simulink model "Project_4_Model"  (R2024b)
settings: Solver=ode4  StartTime=0.0  StopTime=3600  FixedStep=time_step  RelTol=1e-3
undefined symbols (not defined in the file or in its folder): datBat, datCar, datMotor
settings Model: SimulationMode=accelerator  Creator=andis  LastModifiedBy=tyler

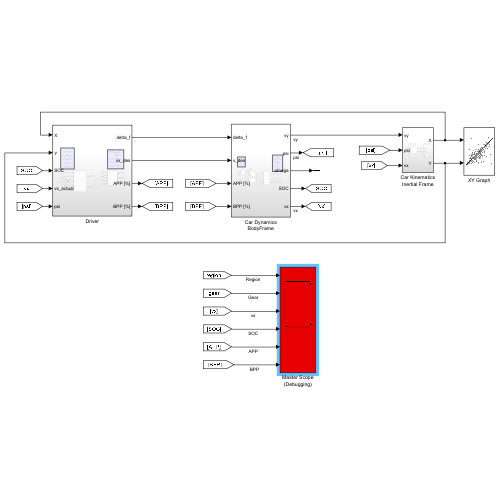
[thumbnail: Simulink's stored preview of the top-level diagram]
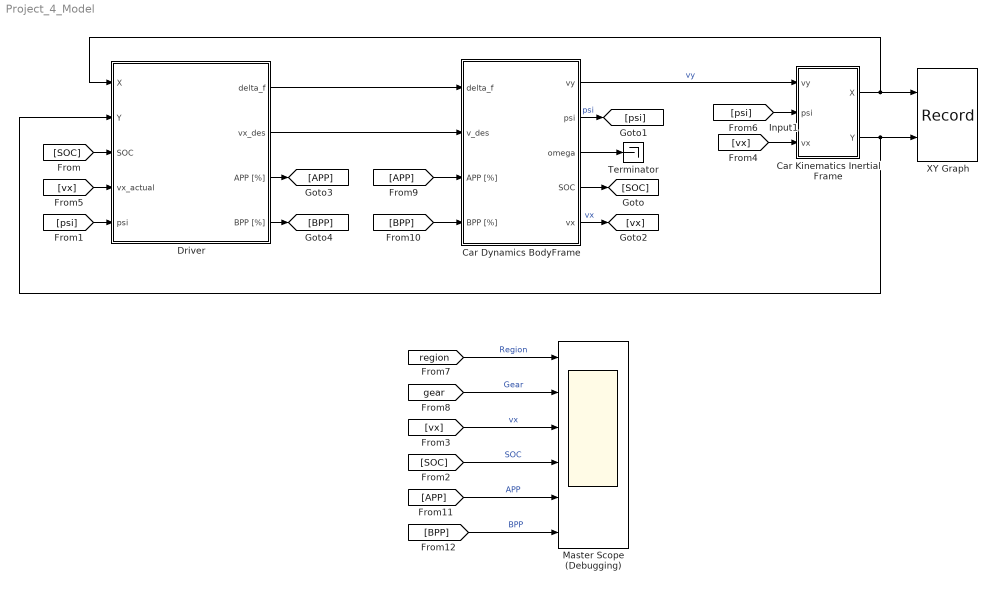
== system Project_4_Model ==
  Input1 : Inport
  Car Dynamics BodyFrame : Subsystem
  Car Kinematics Inertial Frame : Subsystem
  Driver : Subsystem
  Master Scope (Debugging) : Scope  NumInputPorts=6
  Terminator : Terminator
  XY Graph : Record  FileSettingsInternal="{\"entries\":[{\"content\":{\"excelSettings\":{\"content\":{},\"type\":\"Streamout.ExcelSettings\"}},\"type\":\"Streamout.FileSettingStorage\",\"uuid\":\"\"}],\"packageUris\":[\"http:\\/\\/schema.mathworks.com\\/mf0\\/streamout_blocks\\/R2020a\"],\"version\":\"1.0\"}"  Layout=[1 1]  SignalsInternal="{\"entries\":[{\"content\":{\"signals\":[{\"content\":{\"blockPath\":[],\"dimensions\":[1],\"domain\":\"\",\"lineColor\":\"#64d413\",\"lineWidth\":2,\"plots\":[ 1 ],\"port\":1,\"sid\":[\"\"],\"signalID\":1,\"signalName\":\"Car Kinematics\\nInertial Frame:1\"},\"type\":\"RecordBlkView.Signal\",\"uuid\":\"\"},{\"content\":{\"blockPath\":[],\"dimensions\":[1],\"domain\":\"\",\"lineColor\":\"#ff13a6\",\"lineWidth\":2,\"plots\":[ 1 ],\"port\":2,\"sid\":[\"\"],\"signalID\":2,\"signalName\":\"Car Kinematics\\nInertial Frame:2\"},\"type\":\"RecordBlkView.Signal\",\"uuid\":\"\"}]},\"type\":\"RecordBlkView.InputSignals\",\"uuid\":\"\"}],\"packageUris\":[\"http:\\/\\/schema.mathworks.com\\/mf0\\/streamout_blocks\\/R2020a\"],\"version\":\"1.0\"}"  VisualizationBindings="{\"xyplotplugin\":{\"info\":[{\"series\":[{\"bindingParametersList\":[{\"parameter\":\"X-Axis\",\"signalID\":1,\"signalName\":\"Car Kinematics\\nInertial Frame:1\"},{\"parameter\":\"Y-Axis\",\"signalID\":2,\"signalName\":\"Car Kinematics\\nInertial Frame:2\"}],\"seriesID\":0}],\"subplotID\":1}]}}"  CompatibilityTag=XY
  wires:
  Driver/1(delta_f) -> Car Dynamics BodyFrame/1(delta_f)
  Driver/2(vx_des) -> Car Dynamics BodyFrame/2(v_des)
  Car Dynamics BodyFrame/1(vy) -> Car Kinematics Inertial Frame/1(vy)  "vy"
  Car Kinematics Inertial Frame/1(X) -> XY Graph/1, Driver/1(X)
  Car Kinematics Inertial Frame/2(Y) -> Driver/2(Y), XY Graph/2
  Car Dynamics BodyFrame/3(omega) -> Terminator/1
  Car Dynamics BodyFrame/4(SOC) -> [SOC]
  [SOC] -> Driver/3(SOC)
  [psi] -> Driver/5(psi)
  Car Dynamics BodyFrame/2(psi) -> [psi]  "psi"
  [SOC] -> Master Scope (Debugging)/4  "SOC"
  [vx] -> Master Scope (Debugging)/3  "vx"
  [region] -> Master Scope (Debugging)/1  "Region"
  Car Dynamics BodyFrame/5(vx) -> [vx]  "vx"
  [vx] -> Car Kinematics Inertial Frame/3(vx)
  [vx] -> Driver/4(vx_actual)
  [psi] -> Car Kinematics Inertial Frame/2(psi)
  [gear] -> Master Scope (Debugging)/2  "Gear"
  Driver/3(APP [%]) -> [APP]
  Driver/4(BPP [%]) -> [BPP]
  [APP] -> Car Dynamics BodyFrame/3(APP [%])
  [BPP] -> Car Dynamics BodyFrame/4(BPP [%])
  [APP] -> Master Scope (Debugging)/5  "APP"
  [BPP] -> Master Scope (Debugging)/6  "BPP"

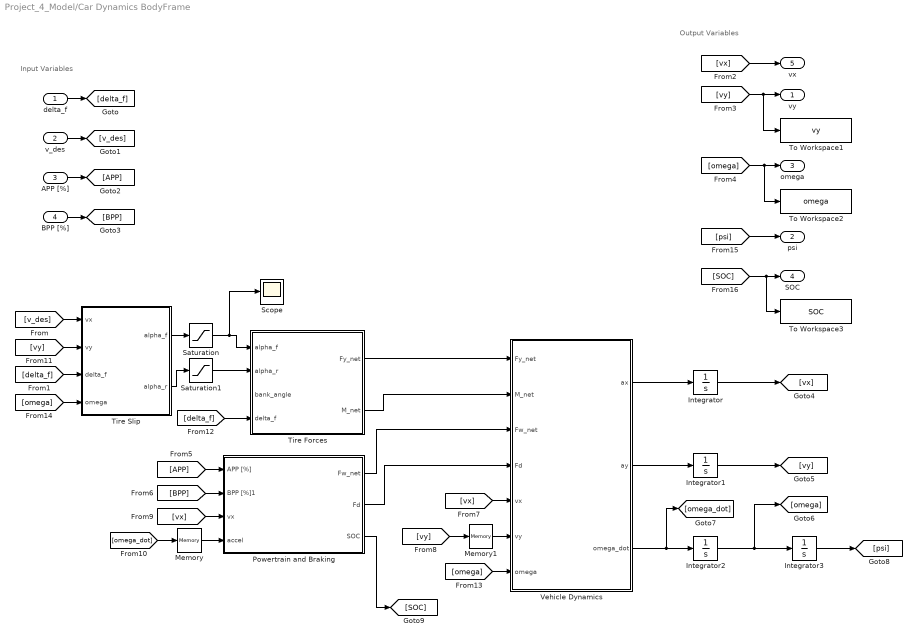
== system Project_4_Model/Car Dynamics BodyFrame ==
  note: Output Variables
  note: Input Variables
  delta_f : Inport
  v_des : Inport  Port=2
  APP [%] : Inport  Port=3
  BPP [%] : Inport  Port=4
  Integrator{,1..3} (4 alike) : Integrator
  Memory : Memory
  Memory1 : Memory
  Powertrain and Braking : Subsystem
  Saturation : Saturate
  Saturation1 : Saturate
  Scope : Scope
  Tire Forces : MATLAB Function  TreatAsAtomicUnit=on
  Tire Slip : MATLAB Function  TreatAsAtomicUnit=on
  To Workspace1 : ToWorkspace  VariableName=vy  SaveFormat=Timeseries  SampleTime=-1
  To Workspace2 : ToWorkspace  VariableName=omega  SaveFormat=Timeseries  SampleTime=-1
  To Workspace3 : ToWorkspace  VariableName=SOC  SaveFormat=Timeseries  SampleTime=-1
  Vehicle Dynamics : MATLAB Function  TreatAsAtomicUnit=on
  vy : Outport
  psi : Outport  Port=2
  omega : Outport  Port=3
  SOC : Outport  Port=4
  vx : Outport  Port=5
  wires:
  Tire Forces/1(Fy_net) -> Vehicle Dynamics/1(Fy_net)
  Tire Forces/2(M_net) -> Vehicle Dynamics/2(M_net)
  delta_f/1 -> [delta_f]
  v_des/1 -> [v_des]
  APP [%]/1 -> [APP]
  BPP [%]/1 -> [BPP]
  [v_des] -> Tire Slip/1(vx)
  [delta_f] -> Tire Slip/3(delta_f)
  Vehicle Dynamics/1(ax) -> Integrator/1
  Vehicle Dynamics/2(ay) -> Integrator1/1
  Vehicle Dynamics/3(omega_dot) -> Integrator2/1, [omega_dot]
  Integrator/1 -> [vx]
  Integrator1/1 -> [vy]
  Integrator2/1 -> [omega], Integrator3/1
  [vx] -> vx/1
  [vy] -> vy/1, To Workspace1/1
  [omega] -> To Workspace2/1, omega/1
  [BPP] -> Powertrain and Braking/2(BPP [%]1)
  [APP] -> Powertrain and Braking/1(APP [%])
  Powertrain and Braking/1(Fw_net) -> Vehicle Dynamics/3(Fw_net)
  Powertrain and Braking/2(Fd) -> Vehicle Dynamics/4(Fd)
  [vx] -> Vehicle Dynamics/5(vx)
  [vx] -> Powertrain and Braking/3(vx)
  [omega_dot] -> Memory/1
  [vy] -> Tire Slip/2(vy)
  [delta_f] -> Tire Forces/4(delta_f)
  Tire Slip/2(alpha_r) -> Saturation1/1
  Tire Slip/1(alpha_f) -> Saturation/1
  Saturation/1 -> Scope/1, Tire Forces/1(alpha_f)
  Saturation1/1 -> Tire Forces/2(alpha_r)
  [omega] -> Vehicle Dynamics/7(omega)
  [omega] -> Tire Slip/4(omega)
  [psi] -> psi/1
  [SOC] -> To Workspace3/1, SOC/1
  Powertrain and Braking/3(SOC) -> [SOC]
  Memory/1 -> Powertrain and Braking/4(accel)
  Integrator3/1 -> [psi]
  Memory1/1 -> Vehicle Dynamics/6(vy)
  [vy] -> Memory1/1

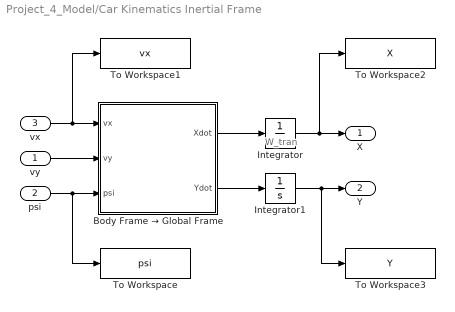
== system Project_4_Model/Car Kinematics Inertial Frame ==
  note: W_tran
  vy : Inport
  psi : Inport  Port=2
  vx : Inport  Port=3
  Body Frame → Global Frame : MATLAB Function  TreatAsAtomicUnit=on
  Integrator : Integrator
  Integrator1 : Integrator
  To Workspace : ToWorkspace  VariableName=psi  SaveFormat=Timeseries  SampleTime=-1
  To Workspace1 : ToWorkspace  VariableName=vx  SaveFormat=Timeseries  SampleTime=-1
  To Workspace2 : ToWorkspace  VariableName=X  SaveFormat=Timeseries  SampleTime=-1
  To Workspace3 : ToWorkspace  VariableName=Y  SaveFormat=Timeseries  SampleTime=-1
  X : Outport
  Y : Outport  Port=2
  wires:
  psi/1 -> To Workspace/1, Body Frame → Global Frame/3(psi)
  Body Frame → Global Frame/1(Xdot) -> Integrator/1
  Body Frame → Global Frame/2(Ydot) -> Integrator1/1
  Integrator1/1 -> To Workspace3/1, Y/1
  Integrator/1 -> To Workspace2/1, X/1
  vx/1 -> To Workspace1/1, Body Frame → Global Frame/1(vx)
  vy/1 -> Body Frame → Global Frame/2(vy)

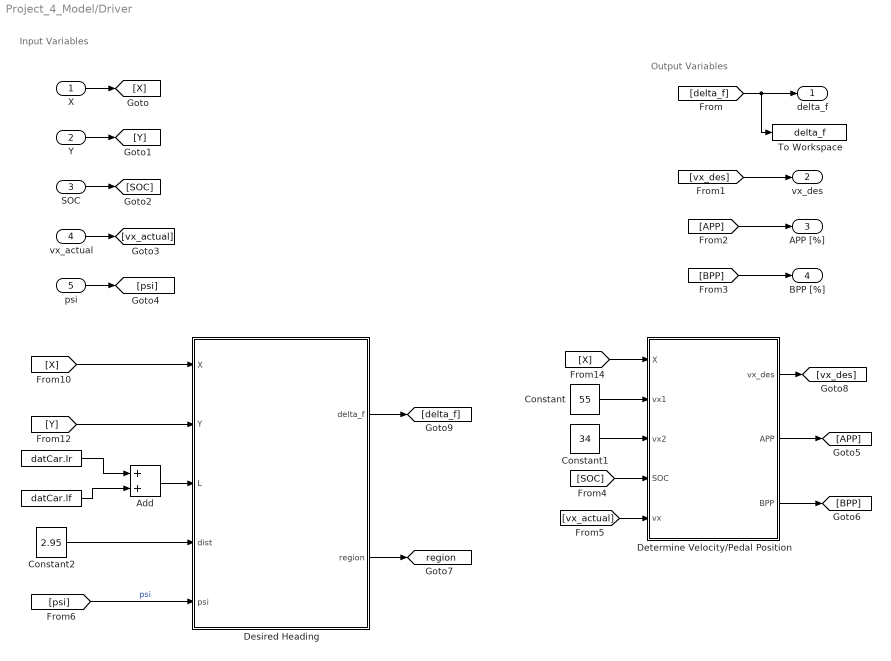
== system Project_4_Model/Driver ==
  note: Output Variables
  note: Input Variables
  X : Inport
  Y : Inport  Port=2
  SOC : Inport  Port=3
  vx_actual : Inport  Port=4
  psi : Inport  Port=5
  " " : Constant  Value=datCar.lr
  "  " : Constant  Value=datCar.lf
  Add : Sum
  Constant : Constant  Value=55
  Constant1 : Constant  Value=34
  Constant2 : Constant  Value=2.95
  Desired Heading : MATLAB Function  TreatAsAtomicUnit=on
  Determine Velocity/Pedal Position : MATLAB Function  TreatAsAtomicUnit=on
  To Workspace : ToWorkspace  VariableName=delta_f  SaveFormat=Timeseries  SampleTime=-1
  delta_f : Outport
  vx_des : Outport  Port=2
  APP [%] : Outport  Port=3
  BPP [%] : Outport  Port=4
  tag scope: region=global
  wires:
  X/1 -> [X]
  Y/1 -> [Y]
  SOC/1 -> [SOC]
  [delta_f] -> To Workspace/1, delta_f/1
  [vx_des] -> vx_des/1
  [APP] -> APP [%]/1
  [BPP] -> BPP [%]/1
  Constant1/1 -> Determine Velocity/Pedal Position/3(vx2)
  Constant/1 -> Determine Velocity/Pedal Position/2(vx1)
  [X] -> Desired Heading/1(X)
  [Y] -> Desired Heading/2(Y)
  [X] -> Determine Velocity/Pedal Position/1(X)
  Determine Velocity/Pedal Position/1(vx_des) -> [vx_des]
  Determine Velocity/Pedal Position/2(APP) -> [APP]
  Determine Velocity/Pedal Position/3(BPP) -> [BPP]
  [SOC] -> Determine Velocity/Pedal Position/4(SOC)
  vx_actual/1 -> [vx_actual]
  [vx_actual] -> Determine Velocity/Pedal Position/5(vx)
  Add/1 -> Desired Heading/3(L)
  "  "/1 -> Add/2
  " "/1 -> Add/1
  Desired Heading/1(delta_f) -> [delta_f]
  Constant2/1 -> Desired Heading/4(dist)
  psi/1 -> [psi]
  [psi] -> Desired Heading/5(psi)  "psi"
  Desired Heading/2(region) -> [region]

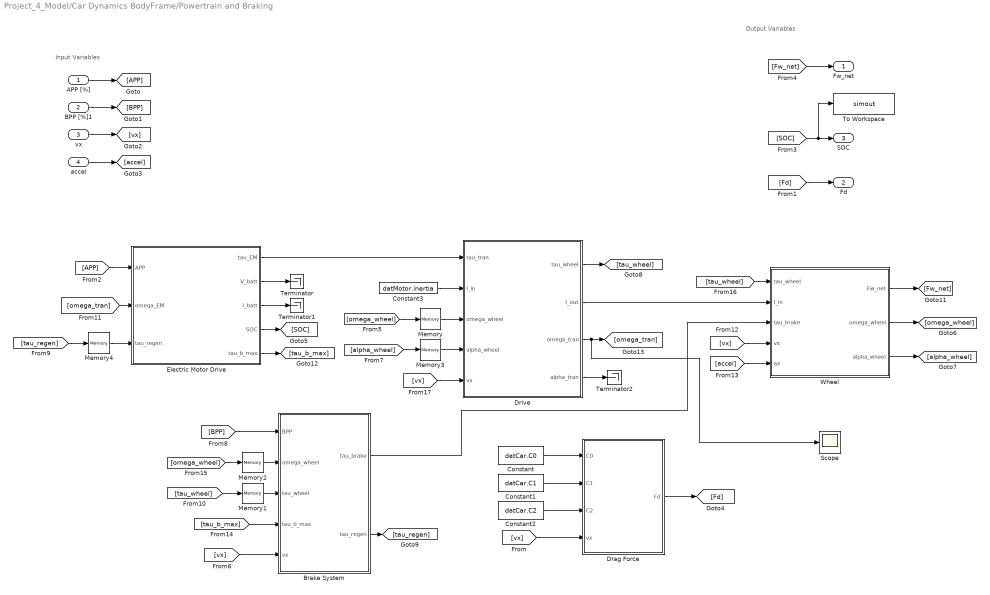
== system Project_4_Model/Car Dynamics BodyFrame/Powertrain and Braking ==
  note: Output Variables
  note: Input Variables
  APP [%] : Inport
  BPP [%]1 : Inport  Port=2
  vx : Inport  Port=3
  accel : Inport  Port=4
  Brake System : Subsystem
  Constant : Constant  Value=datCar.C0
  Constant1 : Constant  Value=datCar.C1
  Constant2 : Constant  Value=datCar.C2
  Constant3 : Constant  Value=datMotor.inertia
  Drag Force : MATLAB Function  TreatAsAtomicUnit=on
  Drive : Subsystem
  Electric Motor Drive : Subsystem
  Memory{,1..4} (5 alike) : Memory
  Scope : Scope
  Terminator : Terminator
  Terminator1 : Terminator
  Terminator2 : Terminator
  To Workspace : ToWorkspace  VariableName=simout  SaveFormat=Timeseries  SampleTime=-1
  Wheel : Subsystem
  Fw_net : Outport
  Fd : Outport  Port=2
  SOC : Outport  Port=3
  wires:
  APP [%]/1 -> [APP]
  BPP [%]1/1 -> [BPP]
  vx/1 -> [vx]
  accel/1 -> [accel]
  Constant/1 -> Drag Force/1(C0)
  Constant1/1 -> Drag Force/2(C1)
  Constant2/1 -> Drag Force/3(C2)
  [vx] -> Drag Force/4(vx)
  Drag Force/1(Fd) -> [Fd]
  [Fd] -> Fd/1
  [APP] -> Electric Motor Drive/1(APP)
  [SOC] -> To Workspace/1, SOC/1
  [Fw_net] -> Fw_net/1
  Electric Motor Drive/4(SOC) -> [SOC]
  Electric Motor Drive/2(V_batt) -> Terminator/1
  Electric Motor Drive/3(I_batt) -> Terminator1/1
  Electric Motor Drive/1(tau_EM) -> Drive/1(tau_tran)
  Wheel/2(omega_wheel) -> [omega_wheel]
  [omega_wheel] -> Memory/1
  [omega_wheel] -> Memory2/1
  Wheel/3(alpha_wheel) -> [alpha_wheel]
  [alpha_wheel] -> Memory3/1
  [BPP] -> Brake System/1(BPP)
  Drive/1(tau_wheel) -> [tau_wheel]
  [tau_wheel] -> Memory1/1
  Drive/2(I_out) -> Wheel/2(I_in)
  Brake System/1(tau_brake) -> Wheel/3(tau_brake)
  Drive/4(alpha_tran) -> Terminator2/1
  Drive/3(omega_tran) -> Scope/1, [omega_tran]
  [omega_tran] -> Electric Motor Drive/2(omega_EM)
  [vx] -> Wheel/4(vx)
  Wheel/1(Fw_net) -> [Fw_net]
  [accel] -> Wheel/5(ax)
  Constant3/1 -> Drive/2(I_in)
  [tau_b_max] -> Brake System/4(tau_b_max)
  Electric Motor Drive/5(tau_b_max) -> [tau_b_max]
  [vx] -> Brake System/5(vx)
  Brake System/2(tau_regen) -> [tau_regen]
  [tau_regen] -> Memory4/1
  Memory/1 -> Drive/3(omega_wheel)
  Memory1/1 -> Brake System/3(tau_wheel)
  Memory2/1 -> Brake System/2(omega_wheel)
  Memory3/1 -> Drive/4(alpha_wheel)
  Memory4/1 -> Electric Motor Drive/3(tau_regen)
  [tau_wheel] -> Wheel/1(tau_wheel)
  [vx] -> Drive/5(vx)

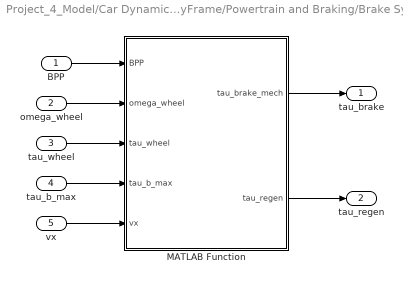
== system Project_4_Model/Car Dynamics BodyFrame/Powertrain and Braking/Brake System ==
  BPP : Inport
  omega_wheel : Inport  Port=2
  tau_wheel : Inport  Port=3
  tau_b_max : Inport  Port=4
  vx : Inport  Port=5
  MATLAB Function : MATLAB Function  TreatAsAtomicUnit=on
  tau_brake : Outport
  tau_regen : Outport  Port=2
  wires:
  BPP/1 -> MATLAB Function/1(BPP)
  omega_wheel/1 -> MATLAB Function/2(omega_wheel)
  tau_wheel/1 -> MATLAB Function/3(tau_wheel)
  tau_b_max/1 -> MATLAB Function/4(tau_b_max)
  MATLAB Function/1(tau_brake_mech) -> tau_brake/1
  vx/1 -> MATLAB Function/5(vx)
  MATLAB Function/2(tau_regen) -> tau_regen/1

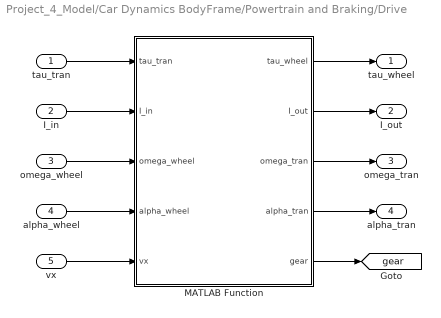
== system Project_4_Model/Car Dynamics BodyFrame/Powertrain and Braking/Drive ==
  tau_tran : Inport
  I_in : Inport  Port=2
  omega_wheel : Inport  Port=3
  alpha_wheel : Inport  Port=4
  vx : Inport  Port=5
  MATLAB Function : MATLAB Function  TreatAsAtomicUnit=on
  tau_wheel : Outport
  I_out : Outport  Port=2
  omega_tran : Outport  Port=3
  alpha_tran : Outport  Port=4
  tag scope: gear=global
  wires:
  tau_tran/1 -> MATLAB Function/1(tau_tran)
  I_in/1 -> MATLAB Function/2(I_in)
  omega_wheel/1 -> MATLAB Function/3(omega_wheel)
  alpha_wheel/1 -> MATLAB Function/4(alpha_wheel)
  MATLAB Function/1(tau_wheel) -> tau_wheel/1
  MATLAB Function/2(I_out) -> I_out/1
  MATLAB Function/3(omega_tran) -> omega_tran/1
  MATLAB Function/4(alpha_tran) -> alpha_tran/1
  MATLAB Function/5(gear) -> [gear]
  vx/1 -> MATLAB Function/5(vx)

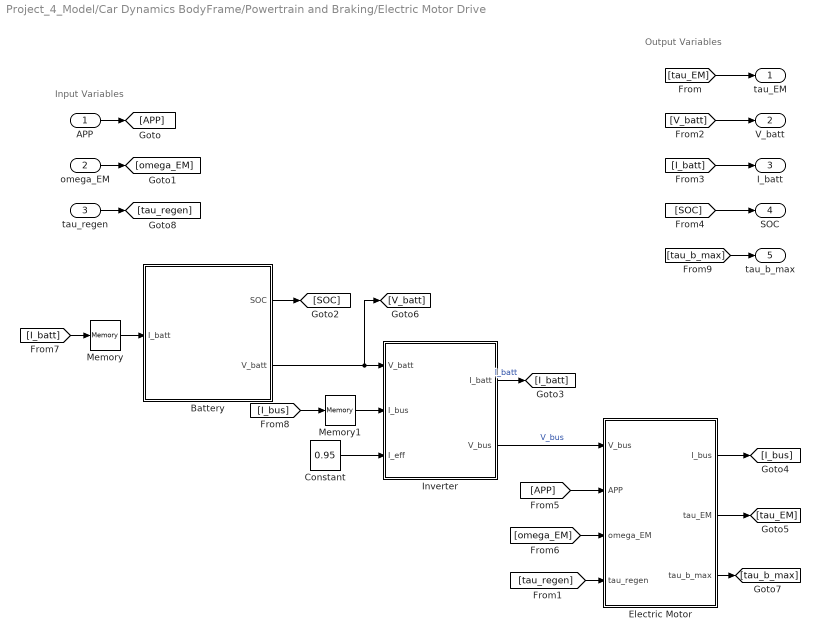
== system Project_4_Model/Car Dynamics BodyFrame/Powertrain and Braking/Electric Motor Drive ==
  note: Output Variables
  note: Input Variables
  APP : Inport
  omega_EM : Inport  Port=2
  tau_regen : Inport  Port=3
  Battery : Subsystem
  Constant : Constant  Value=0.95
  Electric Motor : Subsystem
  Inverter : MATLAB Function  TreatAsAtomicUnit=on
  Memory : Memory
  Memory1 : Memory
  tau_EM : Outport
  V_batt : Outport  Port=2
  I_batt : Outport  Port=3
  SOC : Outport  Port=4
  tau_b_max : Outport  Port=5
  wires:
  APP/1 -> [APP]
  omega_EM/1 -> [omega_EM]
  [tau_EM] -> tau_EM/1
  [V_batt] -> V_batt/1
  [I_batt] -> I_batt/1
  [SOC] -> SOC/1
  Battery/2(V_batt) -> [V_batt], Inverter/1(V_batt)
  Inverter/2(V_bus) -> Electric Motor/1(V_bus)  "V_bus"
  Constant/1 -> Inverter/3(I_eff)
  Battery/1(SOC) -> [SOC]
  [APP] -> Electric Motor/2(APP)
  [omega_EM] -> Electric Motor/3(omega_EM)
  Inverter/1(I_batt) -> [I_batt]  "I_batt"
  [I_batt] -> Memory/1
  [I_bus] -> Memory1/1
  Electric Motor/1(I_bus) -> [I_bus]
  Electric Motor/2(tau_EM) -> [tau_EM]
  [tau_b_max] -> tau_b_max/1
  Electric Motor/3(tau_b_max) -> [tau_b_max]
  tau_regen/1 -> [tau_regen]
  [tau_regen] -> Electric Motor/4(tau_regen)
  Memory/1 -> Battery/1(I_batt)
  Memory1/1 -> Inverter/2(I_bus)

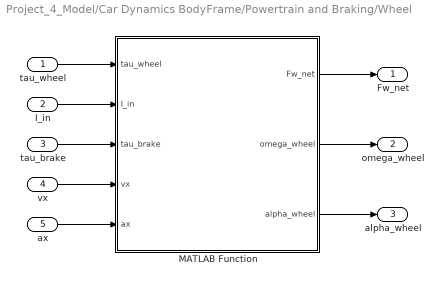
== system Project_4_Model/Car Dynamics BodyFrame/Powertrain and Braking/Wheel ==
  tau_wheel : Inport
  I_in : Inport  Port=2
  tau_brake : Inport  Port=3
  vx : Inport  Port=4
  ax : Inport  Port=5
  MATLAB Function : MATLAB Function  TreatAsAtomicUnit=on
  Fw_net : Outport
  omega_wheel : Outport  Port=2
  alpha_wheel : Outport  Port=3
  wires:
  MATLAB Function/1(Fw_net) -> Fw_net/1
  MATLAB Function/2(omega_wheel) -> omega_wheel/1
  MATLAB Function/3(alpha_wheel) -> alpha_wheel/1
  ax/1 -> MATLAB Function/5(ax)
  vx/1 -> MATLAB Function/4(vx)
  tau_brake/1 -> MATLAB Function/3(tau_brake)
  I_in/1 -> MATLAB Function/2(I_in)
  tau_wheel/1 -> MATLAB Function/1(tau_wheel)

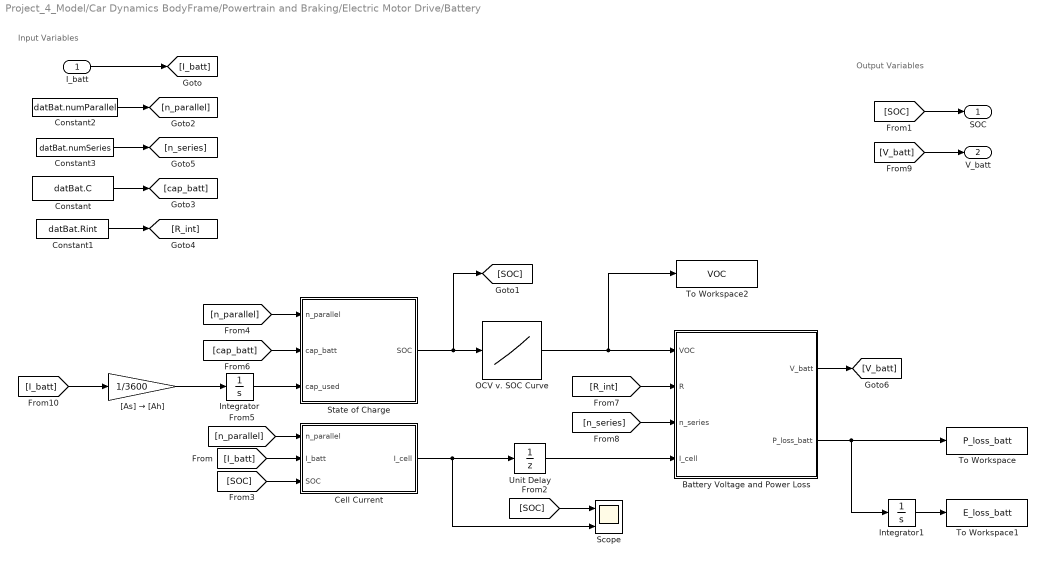
== system Project_4_Model/Car Dynamics BodyFrame/Powertrain and Braking/Electric Motor Drive/Battery ==
  note: Output Variables
  note: Input Variables
  I_batt : Inport
  Battery Voltage and Power Loss : MATLAB Function  TreatAsAtomicUnit=on
  Cell Current : MATLAB Function  TreatAsAtomicUnit=on
  Constant : Constant  Value=datBat.C
  Constant1 : Constant  Value=datBat.Rint
  Constant2 : Constant  Value=datBat.numParallel
  Constant3 : Constant  Value=datBat.numSeries
  Integrator : Integrator
  Integrator1 : Integrator
  OCV v. SOC Curve : Lookup_n-D  NumberOfTableDimensions=1  BreakpointsForDimension1=datBat.SOC  Table=datBat.OCV  InternalRulePriority=Speed  RndMeth=Simplest  mask{BatteryData=datBat}
  Scope : Scope  NumInputPorts=2
  State of Charge : MATLAB Function  TreatAsAtomicUnit=on
  To Workspace : ToWorkspace  VariableName=P_loss_batt  SaveFormat=Timeseries  SampleTime=-1
  To Workspace1 : ToWorkspace  VariableName=E_loss_batt  SaveFormat=Timeseries  SampleTime=-1
  To Workspace2 : ToWorkspace  VariableName=VOC  SaveFormat=Timeseries  SampleTime=-1
  Unit Delay : UnitDelay  SampleTime=-1  HasFrameUpgradeWarning=on
  "[As] → [Ah]" : Gain  Gain=1/3600
  SOC : Outport
  V_batt : Outport  Port=2
  wires:
  Battery Voltage and Power Loss/2(P_loss_batt) -> To Workspace/1, Integrator1/1
  Integrator1/1 -> To Workspace1/1
  OCV v. SOC Curve/1 -> Battery Voltage and Power Loss/1(VOC), To Workspace2/1
  Unit Delay/1 -> Battery Voltage and Power Loss/4(I_cell)
  Cell Current/1(I_cell) -> Unit Delay/1, Scope/2
  I_batt/1 -> [I_batt]
  [I_batt] -> Cell Current/2(I_batt)
  [SOC] -> Cell Current/3(SOC)
  [SOC] -> Scope/1
  State of Charge/1(SOC) -> OCV v. SOC Curve/1, [SOC]
  [SOC] -> SOC/1
  [n_parallel] -> State of Charge/1(n_parallel)
  [n_parallel] -> Cell Current/1(n_parallel)
  Constant2/1 -> [n_parallel]
  Constant/1 -> [cap_batt]
  [cap_batt] -> State of Charge/2(cap_batt)
  Constant1/1 -> [R_int]
  [R_int] -> Battery Voltage and Power Loss/2(R)
  Constant3/1 -> [n_series]
  [n_series] -> Battery Voltage and Power Loss/3(n_series)
  [V_batt] -> V_batt/1
  Battery Voltage and Power Loss/1(V_batt) -> [V_batt]
  Integrator/1 -> State of Charge/3(cap_used)
  "[As] → [Ah]"/1 -> Integrator/1
  [I_batt] -> "[As] → [Ah]"/1

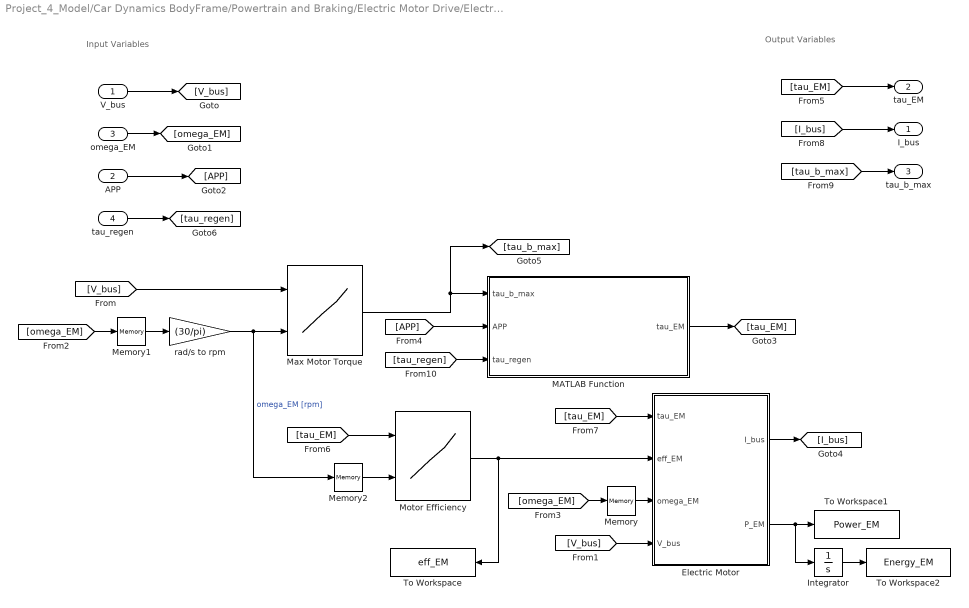
== system Project_4_Model/Car Dynamics BodyFrame/Powertrain and Braking/Electric Motor Drive/Electric Motor ==
  note: Output Variables
  note: Input Variables
  V_bus : Inport
  APP : Inport  Port=2
  omega_EM : Inport  Port=3
  tau_regen : Inport  Port=4
  Electric Motor : MATLAB Function  TreatAsAtomicUnit=on
  Integrator : Integrator
  MATLAB Function : MATLAB Function  TreatAsAtomicUnit=on
  Max Motor Torque : Lookup_n-D  BreakpointsForDimension1=datMotor.vbus  BreakpointsForDimension2=datMotor.rpm  Table=datMotor.maxtorque  InternalRulePriority=Speed  RndMeth=Simplest  mask{BatteryData=datMotor}
      settings: InputPortMap=u0,u1
  Memory : Memory
  Memory1 : Memory
  Memory2 : Memory
  Motor Efficiency : Lookup_n-D  BreakpointsForDimension1=datMotor.eta_torque  BreakpointsForDimension2=datMotor.eta_speed  Table=datMotor.eta_val  InternalRulePriority=Speed  RndMeth=Simplest  mask{MotorEfficiency=datMotor}
      settings: InputPortMap=u0,u1
  To Workspace : ToWorkspace  VariableName=eff_EM  SaveFormat=Timeseries  SampleTime=-1
  To Workspace1 : ToWorkspace  VariableName=Power_EM  SaveFormat=Timeseries  SampleTime=-1
  To Workspace2 : ToWorkspace  VariableName=Energy_EM  SaveFormat=Timeseries  SampleTime=-1
  rad/s to rpm : Gain  Gain=(30/pi)
  I_bus : Outport
  tau_EM : Outport  Port=2
  tau_b_max : Outport  Port=3
  wires:
  Motor Efficiency/1 -> Electric Motor/2(eff_EM), To Workspace/1
  Max Motor Torque/1 -> [tau_b_max], MATLAB Function/1(tau_b_max)
  Integrator/1 -> To Workspace2/1
  rad/s to rpm/1 -> Max Motor Torque/2, Memory2/1  "omega_EM [rpm]"
  Electric Motor/2(P_EM) -> Integrator/1, To Workspace1/1
  [V_bus] -> Electric Motor/4(V_bus)
  [V_bus] -> Max Motor Torque/1
  V_bus/1 -> [V_bus]
  [omega_EM] -> Memory/1
  omega_EM/1 -> [omega_EM]
  [omega_EM] -> Memory1/1
  APP/1 -> [APP]
  [APP] -> MATLAB Function/2(APP)
  [tau_EM] -> tau_EM/1
  [tau_EM] -> Motor Efficiency/1
  [tau_EM] -> Electric Motor/1(tau_EM)
  [I_bus] -> I_bus/1
  Electric Motor/1(I_bus) -> [I_bus]
  [tau_b_max] -> tau_b_max/1
  tau_regen/1 -> [tau_regen]
  [tau_regen] -> MATLAB Function/3(tau_regen)
  Memory/1 -> Electric Motor/3(omega_EM)
  Memory1/1 -> rad/s to rpm/1
  Memory2/1 -> Motor Efficiency/2
  MATLAB Function/1(tau_EM) -> [tau_EM]

== matlab function Project_4_Model/Car Dynamics BodyFrame/Powertrain and Braking/Electric Motor Drive/Electric Motor/MATLAB Function ==
  data: tau_b_max input; APP input; tau_EM output; tau_regen input
function tau_EM = fcn(tau_b_max, APP, tau_regen)

    tau_EM = (tau_b_max * APP) - tau_regen;
    tau_EM = max(-tau_b_max, min(tau_EM, tau_b_max));
end

== matlab function Project_4_Model/Car Dynamics BodyFrame/Powertrain and Braking/Drive/MATLAB Function ==
  data: tau_tran input; tau_wheel output; I_in input; omega_wheel input; alpha_wheel input; I_out output; omega_tran output; alpha_tran output; datCar parameter; gear output; vx input
function [tau_wheel, I_out, omega_tran, alpha_tran, gear] = fcn(tau_tran, I_in, omega_wheel, alpha_wheel, datCar, vx)
% Description:
    % Models drivetrain torque and speed transfer to the wheels
% Inputs:
    % tau_tran - transmission output torque [N-m]
    % I_in - motor inertia [kg-m^2]
    % omega_wheel - wheel speed [rad/s]
    % alpha_wheel - wheel acceleration [rad/s^2]
% Outputs:
    % tau_wheel - wheel torque [N-m]
    % I_out - effective inertia at wheels [kg-m^2]
    % omega_tran - transmission shaft speed [rad/s]
    % alpha_tran - transmission shaft acceleration [rad/s^2]

    % Gear ratio selected based on wheel speed
    if vx < 20
        GR = datCar.gearRatio1; % 1st gear
        gear = 1;
    elseif vx < 40
        GR = datCar.gearRatio2; % 2nd gear
        gear = 2;
    else
        GR = datCar.gearRatio3; % 3rd gear
        gear = 3;
    end

    % Torque multipliplication
    tau_wheel = tau_tran * GR;

    % Reflected inertia at wheel side
    I_out = I_in * GR^2;

    % Transmission speed and acceleration (upstream)
    omega_tran = omega_wheel * GR;
    alpha_tran = alpha_wheel * GR;
end

== matlab function Project_4_Model/Car Dynamics BodyFrame/Powertrain and Braking/Electric Motor Drive/Battery/Cell Current ==
  data: n_parallel input; I_batt input; I_cell output; SOC input
function I_cell = fcn(n_parallel, I_batt, SOC)
% Description:
    % Calculates the current through each individual cell
% Inputs:
    % n_parallel - number of parallel cells
    % I_batt - total battery current draw [A]
    % SOC - state of charge (0 to 1)
% Outputs:
    % I_cell - current through a single cell [A]

    if SOC < 0.05
        I_cell = 0;
    else
        I_cell = I_batt / n_parallel;
    end
end

== matlab function Project_4_Model/Car Dynamics BodyFrame/Powertrain and Braking/Electric Motor Drive/Battery/Battery Voltage and Power Loss ==
  data: VOC input; V_batt output; R input; n_series input; P_loss_batt output; I_cell input
function [V_batt, P_loss_batt] = fcn(VOC, R, n_series, I_cell)
% Description:
    % Calculates total battery pack voltage and internal power loss
% Inputs:
    % VOC - open circuit voltage of a single cell [V]
    % R - internal resistance of a single cell [Ohm]
    % n_series - number of series-connected cells
    % I_cell - current through each cell [A]
% Outputs:
    % V_batt - total battery voltage [V]
    % P_loss_batt - total internal power loss [W]

    V_cell = VOC - I_cell * R; % terminal voltage of each cell
    V_batt = n_series * V_cell;

    P_loss_cell = (I_cell^2) * R;
    P_loss_batt = P_loss_cell * n_series; % total loss scales with series cells
end

== matlab function Project_4_Model/Car Dynamics BodyFrame/Powertrain and Braking/Electric Motor Drive/Battery/State of Charge ==
  data: n_parallel input; cap_batt input; SOC output; cap_used input
function SOC = fcn(n_parallel, cap_batt, cap_used)
% Description:
    % Calculates updated state of charge
% Inputs:
    % n_parallel - number of parallel cells
    % cap_batt - capacity of a single cell [Ah]
    % cap_used - total capacity used from the pack so far [Ah]
% Outputs:
    % SOC - updated state of charge (0 to 1)

    if cap_used == 0  % start with 80% battery
        SOC = 0.8;
    else
        total_cap = n_parallel * cap_batt;
        SOC = 0.8 - (cap_used / total_cap);
        SOC = max(0, min(1, SOC)); % clamp to (0, 1)
    end
end

== matlab function Project_4_Model/Car Dynamics BodyFrame/Powertrain and Braking/Electric Motor Drive/Electric Motor/Electric Motor ==
  data: tau_EM input; eff_EM input; omega_EM input; V_bus input; I_bus output; P_EM output
function [I_bus, P_EM] = fcn(tau_EM,  eff_EM, omega_EM,V_bus)
% Description:
    % Calculates motor power output and bus current draw
% Inputs:
    % tau_EM - motor torque [N-m]
    % eff_EM - motor efficiency (0 to 1)
    % omega_EM - motor speed [rad/s]
    % V_bus - DC bus voltage [V]
% Outputs:
    % I_bus - current draw from DC bus [A]
    % P_EM - mechanical power output of the motor [W]

    % Protect against divide-by-zero error
    eff_EM = max(0.01, min(1, eff_EM));
    V_bus = max(1e-3, V_bus); 

    % Mechanical output power
    P_EM = tau_EM * omega_EM;

    % Electrical input power to motor
    P_in = P_EM / eff_EM;

    % Bus current draw
    I_bus = P_in / V_bus;
end

== matlab function Project_4_Model/Car Dynamics BodyFrame/Powertrain and Braking/Electric Motor Drive/Inverter ==
  data: V_batt input; I_bus input; I_batt output; V_bus output; I_eff input
function [I_batt, V_bus] = fcn(V_batt, I_bus, I_eff)
% Description:
    % Simulates a basic inverter's behavior
% Inputs:
    % V_batt - battery voltage [V]
    % I_bus - current demand from the motor side [A]
    % I_eff - inverter efficiency (0 to 1)
% Outputs:
    % I_batt - current draw from the battery [A]
    % V_bus - voltage available on the motor side DC bus [V]

    % Protect against divide-by-zero error
    I_eff = max(0.01, min(1, I_eff));

    % Power output to the motor
    P_out = I_bus * (V_batt * I_eff);

    % Bus voltage seen by motor
    V_bus = V_batt * I_eff;

    % Battery current needed to support output power
    I_batt = P_out / V_batt;
end

== matlab function Project_4_Model/Car Dynamics BodyFrame/Powertrain and Braking/Brake System/MATLAB Function ==
  data: BPP input; tau_brake_mech output; omega_wheel input; tau_wheel input; tau_b_max input; vx input; tau_regen output
function [tau_brake_mech, tau_regen] = fcn(BPP, omega_wheel, tau_wheel, tau_b_max, vx)
% Description:
    % Calculates total braking torque based on driver brake pedal input,
    % and splits the torque into a regenerative component and a remaining
    % friction (mechanical) component. Regen contribution ramps up with
    % speed between 5 and 25 [mph], and is limited by the current wheel
    % torque to prevent exceeding available deceleration. Below 5 [mph],
    % only friction braking is used.
% Inputs:
    % BPP - brake pedal position (0 to 1)
    % omega_wheel - wheel speed [rad/s]
    % tau_wheel - current wheel torque [N-m]
    % tau_b_max - max available regen braking torque [N-m]
    % vx - vehicle longitudinal speed [m/s]
% Outputs:
    % tau_brake - friction brake torque applied [N-m]
    % tau_regen - regenerative brake torque applied [N-m]

    % Return zero torque if not braking or wheel is stopped
    if BPP <= 0 || omega_wheel <= 0.1
        tau_brake_mech = 0;
        tau_regen = 0;
        return;
    end

    % Requested braking torque
    tau_des = BPP * tau_b_max;

    % Convert actual speed [m/s] to [mph]
    vx = vx * (3600/1600);

    % Regen factor based on speed
    if vx < 5
        regen = 0;
    elseif vx >= 25
        regen = 0.95;
    else
        regen = 0.95 * (vx - 5) / 20;
    end

    % Requested regen torque (limited by tau_wheel)
    tau_regen = min(regen * tau_des, tau_wheel);

    % Remaining friction braking
    tau_brake_mech = max(tau_des - tau_regen, 0);
end

== matlab function Project_4_Model/Car Dynamics BodyFrame/Powertrain and Braking/Wheel/MATLAB Function ==
  data: tau_wheel input; Fw_net output; I_in input; tau_brake input; vx input; ax input; omega_wheel output; alpha_wheel output; datCar parameter
function [Fw_net, omega_wheel, alpha_wheel] = fcn(tau_wheel, I_in, tau_brake, vx, ax, datCar)
% Description:
    % Calculates net longitudinal force from drive and brake torque
% Inputs:
    % tau_wheel - applied wheel torque [N-m]
    % I_in - rotational inertia at the wheel [kg-m^2]
    % tau_brake - brake torque applied [N-m]
    % vx - vehicle longitudinal speed [m/s]
    % ax - vehicle longitudinal acceleration [m/s^2]
% Outputs:
    % Fw_net - net longitudinal force at the wheel-ground interface [N]
    % omega_wheel - wheel angular velocity [rad/s]
    % alpha_wheel - wheel angular acceleration [rad/s^2]
% Assumptions:
    % Tires are rolling without slip: 
        % omega_wheel = vx / r_tire
    % Net torque is the difference between wheel and brake torque:
        % tau_net = tau_wheel - tau_brake

    r_tire = datCar.radius; % tire radius [m]
    tau_net = tau_wheel - tau_brake; % net torque at the wheel
    
    % Angular velocity from rotational dynamics
    alpha_wheel = tau_net / I_in; 
    % Angular velocity from linear speed (no slip)
    omega_wheel = vx / r_tire;
    % Longitudinal force transmitted at the contact patch
    Fw_net = tau_net / r_tire;
end

== matlab function Project_4_Model/Car Dynamics BodyFrame/Tire Forces ==
  data: alpha_f input; Fy_net output; alpha_r input; bank_angle input; delta_f input; M_net output; datCar parameter
function [Fy_net, M_net] = fcn(alpha_f, alpha_r, bank_angle, delta_f, datCar)
% Description:
    % Computes the net lateral force and net yaw moment acting on the
    % vehicle, accounting for tire slip angles and road bank angle. This is
    % useful in lateral dynamics modeling to determine how much the vehicle
    % will accelerate sideways and rotate (yaw) under combined steering and
    % banking.
% Inputs:
    % alpha_f - front tire slip angle [rad]
    % alpha_r - rear tire slip angle [rad]
    % bank_angle - road bank angle [rad], positive for banking towards the
        % inside of the track
    % delta_f - front wheel steering angle [rad]
% Outputs:
    % Fy_net - net lateral force on the vehicle body [N]
    % M_net - net yaw moment about the vehicle's center of gravity [N-m]

    % Front tire lateral force (wheel frame)
    Fywf_tire = datCar.Calpha_f * alpha_f; 
    % Rear tire lateral force (wheel frame)
    Fywr_tire = datCar.Calpha_r * alpha_r; 
    % Projected front lateral force (vehicle frame)
    Fyf = Fywf_tire * cos(delta_f); % F_bank_f

    Fyr = Fywr_tire; % Rear lateral force remains unchanged (F_bank_r = 0)
    Fy_t = Fyf + Fyr; % Total tire-generated lateral force

    % Add effect of road banking
    Fy_net = datCar.m * datCar.g * tan(bank_angle) + Fy_t / cos(bank_angle);
    % Yaw moment from front and rear lateral forces
    M_net = (Fyf * datCar.lf) - (Fyr * datCar.lr);
end

== matlab function Project_4_Model/Car Dynamics BodyFrame/Tire Slip ==
  data: vx input; alpha_f output; vy input; delta_f input; omega input; alpha_r output; datCar parameter
function [alpha_f, alpha_r] = fcn(vx, vy, delta_f, omega, datCar)
% Description:
    % Computes the front and rear tire slip angles based on the vehicle's
    % current motion and steering input. Slip angles represent the angle
    % between the direction a tire is pointing and the actual direction it
    % is moving which is essential for modeling lateral tire forces in
    % vehicle dynamics.
% Inputs:
    % vx - longitudinal velocity of the vehicle [m/s]
    % vy - lateral velocity of the vehicle [m/s]
    % delta_f - front wheel steering angle [rad]
    % omega - yaw rate of the vehicle [rad/s]
% Outputs:
    % alpha_f - front tire slip angle [rad]
    % alpha_r - rear tire slip angle [rad]
    
    alpha_f = delta_f - atan((vy + (datCar.lf * omega)) / vx);
    alpha_r = - atan((vy - (datCar.lr * omega)) / vx);
end

== matlab function Project_4_Model/Car Dynamics BodyFrame/Vehicle Dynamics ==
  data: Fy_net input; ax output; M_net input; Fw_net input; Fd input; vx input; vy input; omega input; ay output; omega_dot output; datCar parameter
function [ax, ay, omega_dot] = fcn(Fy_net, M_net, Fw_net, Fd, vx, vy, omega, datCar)
% Description:
    % Computes the vehicle's longitudinal, lateral, and yaw acceleration
    % based on net forces and moments. This function is part of a dynamic
    % vehicle model using Newton's Second Law in both translation and
    % rotational forms.
% Inputs:
    % Fy_net - net lateral force on the vehicle [N]
    % M_net - net yaw moment about the vehicle's center of gravity [N-m]
    % Fw_net - net longitudinal (tractive/braking) force on the vehicle [N]
    % Fd - aerodynamic drag force [N]
    % vx - longitudinal velocity of the vehicle [m/s]
    % vy - lateral velocity of the vehicle [m/s]
    % omega - yaw rate of the vehicle [rad/s]
% Outputs:
    % ax - longitudinal acceleration [m/s^2]
    % ay - lateral acceleration [m/s^2]
    % omega_dot - yaw acceleration [rad/s^2]

    % Longitudinal acceleration from drag
    Fx_net = Fw_net - Fd;
    ax = Fx_net / datCar.m;

    % Lateral acceleration from centripetal + force
    ay = (vy * omega) + (Fy_net / datCar.m);

    % Yaw acceleration from net moment and inertia
    omega_dot = M_net / datCar.I;
end

== matlab function Project_4_Model/Car Dynamics BodyFrame/Powertrain and Braking/Drag Force ==
  data: C0 input; Fd output; C1 input; C2 input; vx input
function Fd = fcn(C0, C1, C2, vx)
% Description:
    % Calculates total resistance force acting against the vehicle's
    % motion, including static, rolling, and aerodynamic drag components.
% Inputs:
    % C0 - static friction coefficient [N]
    % C1 - rolling friction coefficient [N-s/m]
    % C2 - aerodynamic drag coefficient [N-s^2/m^2]
    % vx - vehicle longitudinal velocity [m/s]
% Output:
    % Fd - total drag force [N]

    Fd = C0 + C1 * vx + C2 * vx^2;
end

== matlab function Project_4_Model/Car Kinematics Inertial Frame/Body Frame → Global Frame ==
  data: vx input; Xdot output; vy input; psi input; Ydot output
function [Xdot, Ydot] = fcn(vx, vy, psi)
% Description:
    % Transforms the vehicle's body-frame velocities (vx, vy) into global-frame
    % velocities (Xdot, Ydot) using the vehicle's heading angle (psi).
% Inputs:
    % vx - longitudinal velocity in the body frame [m/s]
    % vy - lateral velocity in the body frame [m/s]
    % psi - vehicle heading angle [rad], measured from global x-axis
% Outputs:
    % Xdot - global x-axis velocity [m/s]
    % Ydot - global y-axis velocity [m/s]

    temp = TF(psi) * [vx;vy];
    Xdot = temp(1);
    Ydot = temp(2);

end

function y = TF(psi)
% Description:
    % Helper function that constructs a 2D rotaiton matrix that rotates
    % vectors from the body frame to the global frame based on heading
    % angle (psi)
    
    y = [cos(psi), -sin(psi); sin(psi), cos(psi)];
end

== matlab function Project_4_Model/Driver/Determine Velocity//Pedal Position ==
  data: X input; vx_des output; vx1 input; vx2 input; SOC input; APP output; BPP output; vx input
function [vx_des, APP, BPP] = fcn(X, vx1, vx2, SOC, vx)
% Description:
    % Determines desired speed and pedal commands
% Inputs:
    % X, Y - vehicle position [m]
    % vx - current speed [m/s]
    % SOC - state of charge (0 to 1)
% Outputs:
    % vx_des - desired forward speed [m/s]
    % APP - accelerator pedal position (0 to 1)
    % BPP - brake pedal position (0 to 1)
    
    % Adjust velocity based on position and SOC
    if SOC > 0.2
        if (X >= -50) && (X <= 950) % straight sections
            vx_des = vx1;
        else
            vx_des = vx2;
        end
    else
        vx_des = vx2;
    end

    % Control logic
    error = vx_des - vx;

    if error > 0.5
        APP = min(error / 5, 1);
        BPP = 0;
    elseif error < -0.5
        APP = 0;
        BPP = min(-error / 5, 1);
    else
        APP = 0;
        BPP = 0;
    end
end

== matlab function Project_4_Model/Driver/Desired Heading ==
  data: X input; Y input; L input; delta_f output; dist input; psi input; region output
function [delta_f, region] = fcn(X, Y, L, dist, psi)
% Description:
    % Calculates steering angle to follow the track centerline
% Inputs:
    % X, Y - vehicle position [m]
    % L - vehicle wheelbase [m]
    % dist - lookahead distance [m]
% Outputs:
    % delta_f - front steering angle command [rad]

    % Parameters
    center_right = [900, 200]; % center of right turn
    center_left = [0, 200]; % center of left turn

    % Region 1: Bottom straight
    if (X >= 0 && X < 900) && (Y > -7.5 && Y < 7.5)
        psi_des = 0;  % +X direction
        % dist = 450;
        region = 1;
        alpha = -0.2*wrapToPi(psi_des - psi);

    % Region 2: Right semicircle
    elseif (X >= 900 && X < 1100) && (Y > -7.5 && Y < 407.5)
        dx = X - center_right(1);
        dy = Y - center_right(2);
        theta = atan2(dy, dx);
        psi_des = wrapToPi(theta - pi/2);  % Clockwise tangent
        region = 2;
        alpha = wrapToPi(psi_des - psi);

    % Region 3: Top straight
    elseif (X >= 0 && X < 900) && (Y > 392.5 && Y < 407.5)
        psi_des = 0;  % -X direction
        % dist = 250;
        region = 3;
        alpha = wrapToPi(psi_des - psi);

    % Region 4: Left semicircle
    elseif (X < 0) && (Y > -7.5 && Y < 407.5)
        dx = X - center_left(1);
        dy = Y - center_left(2);
        theta = atan2(dy, dx);
        psi_des = wrapToPi(theta - pi/2);  % Clockwise tangent
        region = 4;
        alpha = wrapToPi(psi_des - psi);
        dist = 4.5;

    else
        % Fallback if position is outside expected bounds
        psi_des = 0;
        region = 0;
        alpha = 0;
    end

    % Compute steering angle using pure pursuit formula
    delta_f = -atan2(2 * L * sin(alpha), dist);
end
